simulink model "Practica_1"  (R2024a)
settings: Solver=VariableStepAuto  StartTime=0.0  StopTime=10.0  RelTol=1e-3
undefined symbols (not defined in the file): g, l1, l2, m1, m2
settings Model: Creator=Kaleb  LastModifiedBy=Kaleb

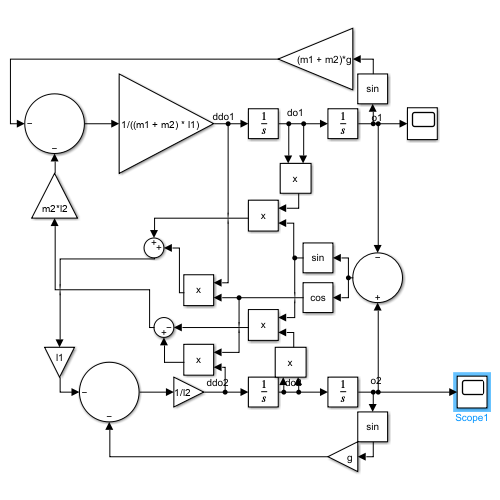
[thumbnail: Simulink's stored preview of the top-level diagram]
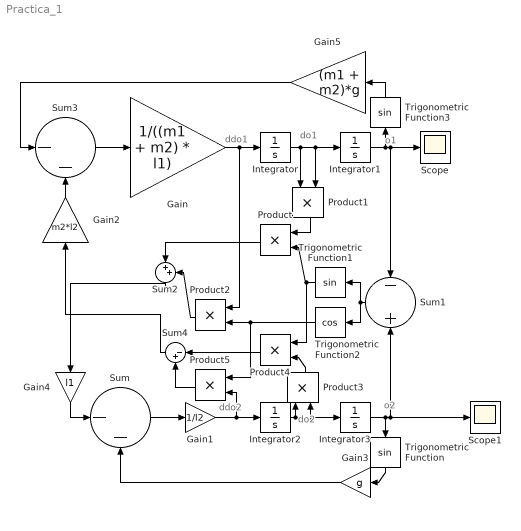
== system Practica_1 ==
  note: ddo2
  note: o2
  note: do2
  note: o1
  note: do1
  note: ddo1
  Gain : Gain  Gain=1/((m1 + m2) * l1)
  Gain1 : Gain  Gain=1/l2
  Gain2 : Gain  Gain=m2*l2
  Gain3 : Gain  Gain=g
  Gain4 : Gain  Gain=l1
  Gain5 : Gain  Gain=(m1 + m2)*g
  Integrator : Integrator
  Integrator1 : Integrator
  Integrator2 : Integrator
  Integrator3 : Integrator  InitialCondition=35
  Product{,1..5} (6 alike) : Product
  Scope : Scope
  Scope1 : Scope
  Sum : Sum  Inputs=|--
  Sum1 : Sum  Inputs=-+
  Sum2 : Sum  Inputs=|++
  Sum3 : Sum  Inputs=|--
  Sum4 : Sum  Inputs=|-+
  Trigonometric Function : Trigonometry
  Trigonometric Function1 : Trigonometry
  Trigonometric Function2 : Trigonometry  Operator=cos
  Trigonometric Function3 : Trigonometry
  wires:
  Integrator/1 -> Product1/1, Product1/2, Integrator1/1
  Gain/1 -> Product2/1, Integrator/1
  Integrator1/1 -> Scope/1, Sum1/1, Trigonometric Function3/1
  Integrator2/1 -> Product3/1, Product3/2, Integrator3/1
  Gain1/1 -> Product5/2, Integrator2/1
  Sum/1 -> Gain1/1
  Integrator3/1 -> Sum1/2, Scope1/1, Trigonometric Function/1
  Trigonometric Function/1 -> Gain3/1
  Sum1/1 -> Trigonometric Function1/1, Trigonometric Function2/1
  Product1/1 -> Product/1
  Trigonometric Function1/1 -> Product4/1, Product/2
  Trigonometric Function2/1 -> Product5/1, Product2/2
  Product2/1 -> Sum2/2
  Product/1 -> Sum2/1
  Sum2/1 -> Gain4/1
  Gain4/1 -> Sum/1
  Gain3/1 -> Sum/2
  Trigonometric Function3/1 -> Gain5/1
  Sum3/1 -> Gain/1
  Gain5/1 -> Sum3/1
  Gain2/1 -> Sum3/2
  Product3/1 -> Product4/2
  Product4/1 -> Sum4/1
  Product5/1 -> Sum4/2
  Sum4/1 -> Gain2/1
